simulink model "EV_Powertrain"  (R2021a)
settings: Solver=FixedStepAuto  StartTime=0.0  StopTime=993  FixedStep=0.5  RelTol=1e-3
values from neighbouring files (symbols this model uses):
  A = 3.8065    [Powertrain_Imports.m]
  B_Voltage = 364.8    [Powertrain_Imports.m]
  Ccap = 33.1    [Powertrain_Imports.m]
  Cd = 0.28    [Powertrain_Imports.m]
  Crf = 0.015    [Powertrain_Imports.m]
  Cv = 3.8    [Powertrain_Imports.m]
  Distance = 4.874    [Powertrain_Imports.m]
  GR = 7.9377    [Powertrain_Imports.m]
  GVM = M+Md    (= 1710.665)    [Powertrain_Imports.m]
  GVW = GVM*g    (= 16781.62365)    [Powertrain_Imports.m]
  ISOC = 1    [Powertrain_Imports.m]
  Neff = 0.89    [Powertrain_Imports.m]
  rho = 1.225    [Powertrain_Imports.m]
  Rw = 0.2032    [Powertrain_Imports.m]
undefined symbols (not defined in the file or in its folder): Motor_controller_eff, Motor_controller_reff, Motor_eff, Motor_reff
settings Model: Creator=mluser  LastModifiedBy=mluser

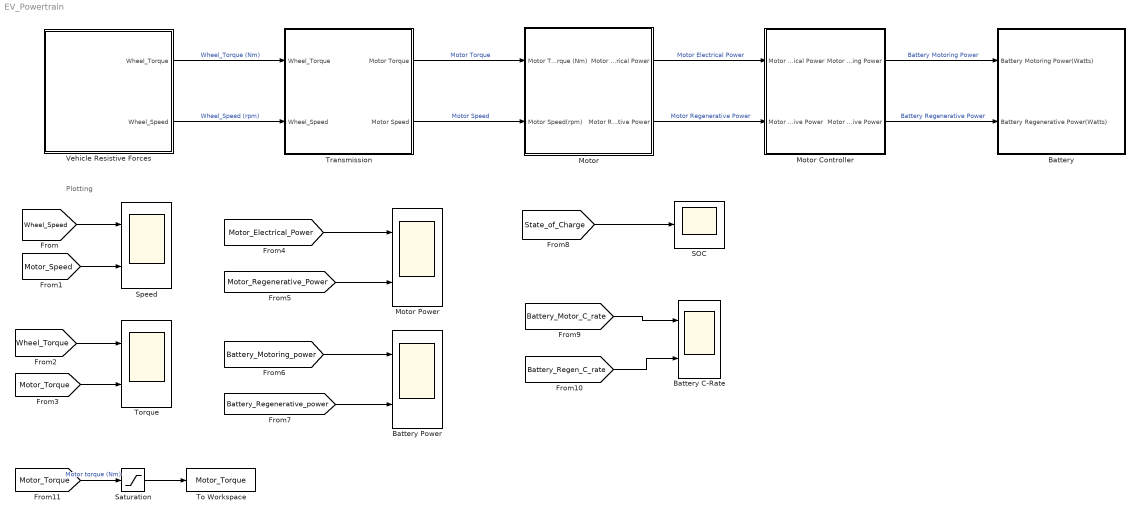
== system EV_Powertrain ==
  note: Plotting
  Battery : Subsystem
  Battery C-Rate : Scope  NumInputPorts=2
  Battery Power : Scope  NumInputPorts=2
  Motor : Subsystem
  Motor Controller : Subsystem
  Motor Power : Scope  NumInputPorts=2
  SOC : Scope
  Saturation : Saturate  UpperLimit=inf  LowerLimit=0
  Speed : Scope  NumInputPorts=2
  To Workspace : ToWorkspace  VariableName=Motor_Torque  SaveFormat=Timeseries  SampleTime=-1
  Torque : Scope  NumInputPorts=2
  Transmission : Subsystem
  Vehicle Resistive Forces : Subsystem
  wires:
  Vehicle Resistive Forces/1(Wheel_Torque) -> Transmission/1(Wheel_Torque)  "Wheel_Torque (Nm)"
  Vehicle Resistive Forces/2(Wheel_Speed) -> Transmission/2(Wheel_Speed)  "Wheel_Speed (rpm)"
  [Wheel_Speed] -> Speed/1
  [Motor_Speed] -> Speed/2
  [Motor_Torque] -> Torque/2
  [Wheel_Torque] -> Torque/1
  Transmission/1(Motor Torque) -> Motor/1(Motor Torque (Nm))  "Motor Torque"
  Transmission/2(Motor Speed) -> Motor/2(Motor Speed(rpm))  "Motor Speed"
  [Motor_Electrical_Power] -> Motor Power/1
  [Motor_Regenerative_Power] -> Motor Power/2
  Motor/1(Motor Electrical Power) -> Motor Controller/1(Motor Electrical Power)  "Motor Electrical Power"
  Motor/2(Motor Regenerative Power) -> Motor Controller/2(Motor Regenerative Power)  "Motor Regenerative Power"
  [Battery_Motoring_power] -> Battery Power/1
  [Battery_Regenerative_power] -> Battery Power/2
  Motor Controller/1(Motor Controller Motoring Power) -> Battery/1(Battery Motoring Power(Watts))  "Battery Motoring Power"
  Motor Controller/2(Motor Controller Regenerative Power) -> Battery/2(Battery Regenerative Power(Watts))  "Battery Regenerative Power"
  [State_of_Charge] -> SOC/1
  [Battery_Regen_C_rate] -> Battery C-Rate/2
  [Battery_Motor_C_rate] -> Battery C-Rate/1
  [Motor_Torque] -> Saturation/1  "Motor torque (Nm)"
  Saturation/1 -> To Workspace/1

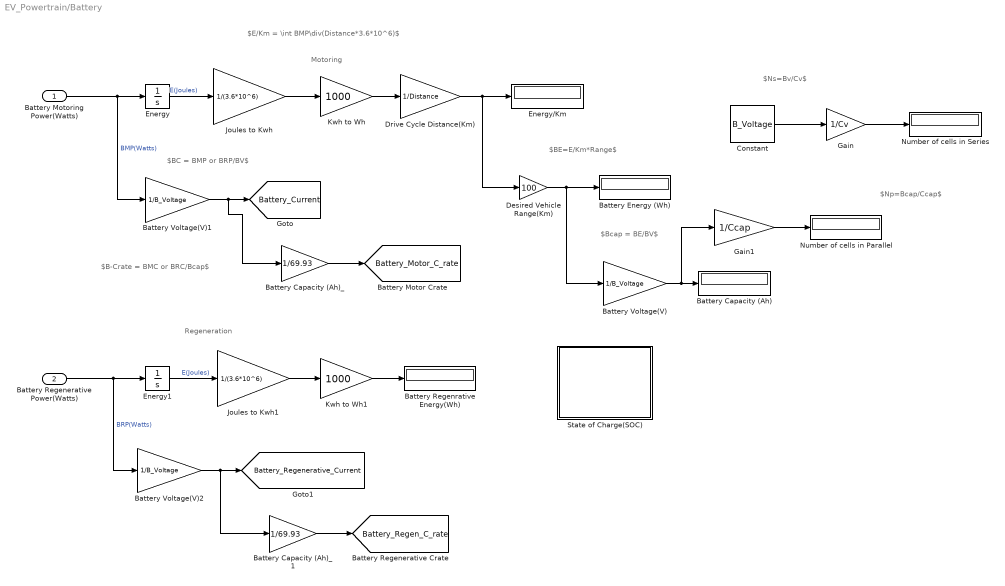
== system EV_Powertrain/Battery ==
  note: $Np=Bcap/Ccap$
  note: $Ns=Bv/Cv$
  note: Regeneration
  note: $B-Crate = BMC or BRC/Bcap$
  note: $BC = BMP or BRP/BV$
  note: $Bcap = BE/BV$
  note: $BE=E/Km*Range$
  note: $E/Km = \int BMP\div(Distance*3.6*10^6)$
  note: Motoring
  Battery Motoring Power(Watts) : Inport
  Battery Regenerative Power(Watts) : Inport  Port=2
  Battery Regenrative Energy(Wh) : Display
  Battery Capacity (Ah) : Display
  Battery Capacity (Ah)_ : Gain  Gain=1/69.93
  Battery Capacity (Ah)_1 : Gain  Gain=1/69.93
  Battery Energy (Wh) : Display
  Battery Voltage(V) : Gain  Gain=1/B_Voltage
  Battery Voltage(V)1 : Gain  Gain=1/B_Voltage
  Battery Voltage(V)2 : Gain  Gain=1/B_Voltage
  Constant : Constant  Value=B_Voltage
  Desired Vehicle Range(Km) : Gain  Gain=100
  Drive Cycle Distance(Km) : Gain  Gain=1/Distance
  Energy : Integrator
  Energy/Km : Display
  Energy1 : Integrator
  Gain : Gain  Gain=1/Cv
  Gain1 : Gain  Gain=1/Ccap
  Joules to Kwh : Gain  Gain=1/(3.6*10^6)
  Joules to Kwh1 : Gain  Gain=1/(3.6*10^6)
  Kwh to Wh : Gain  Gain=1000
  Kwh to Wh1 : Gain  Gain=1000
  Number of cells in Parallel : Display
  Number of cells in Series : Display
  State of Charge(SOC) : Subsystem
  tag scope: Battery_Current=global, Battery_Motor_C_rate=global, Battery_Regen_C_rate=global, Battery_Regenerative_Current=global
  wires:
  Battery Motoring Power(Watts)/1 -> Battery Voltage(V)1/1, Energy/1  "BMP(Watts)"
  Kwh to Wh/1 -> Drive Cycle Distance(Km)/1
  Joules to Kwh/1 -> Kwh to Wh/1
  Energy/1 -> Joules to Kwh/1  "E(Joules)"
  Drive Cycle Distance(Km)/1 -> Desired Vehicle Range(Km)/1, Energy/Km/1
  Desired Vehicle Range(Km)/1 -> Battery Voltage(V)/1, Battery Energy (Wh)/1
  Battery Voltage(V)/1 -> Gain1/1, Battery Capacity (Ah)/1
  Battery Voltage(V)1/1 -> Battery Capacity (Ah)_/1, [Battery_Current]
  Battery Voltage(V)2/1 -> Battery Capacity (Ah)_1/1, [Battery_Regenerative_Current]
  Battery Regenerative Power(Watts)/1 -> Battery Voltage(V)2/1, Energy1/1  "BRP(Watts)"
  Energy1/1 -> Joules to Kwh1/1  "E(Joules)"
  Joules to Kwh1/1 -> Kwh to Wh1/1
  Kwh to Wh1/1 -> Battery Regenrative Energy(Wh)/1
  Battery Capacity (Ah)_/1 -> [Battery_Motor_C_rate]
  Battery Capacity (Ah)_1/1 -> [Battery_Regen_C_rate]
  Constant/1 -> Gain/1
  Gain/1 -> Number of cells in Series/1
  Gain1/1 -> Number of cells in Parallel/1

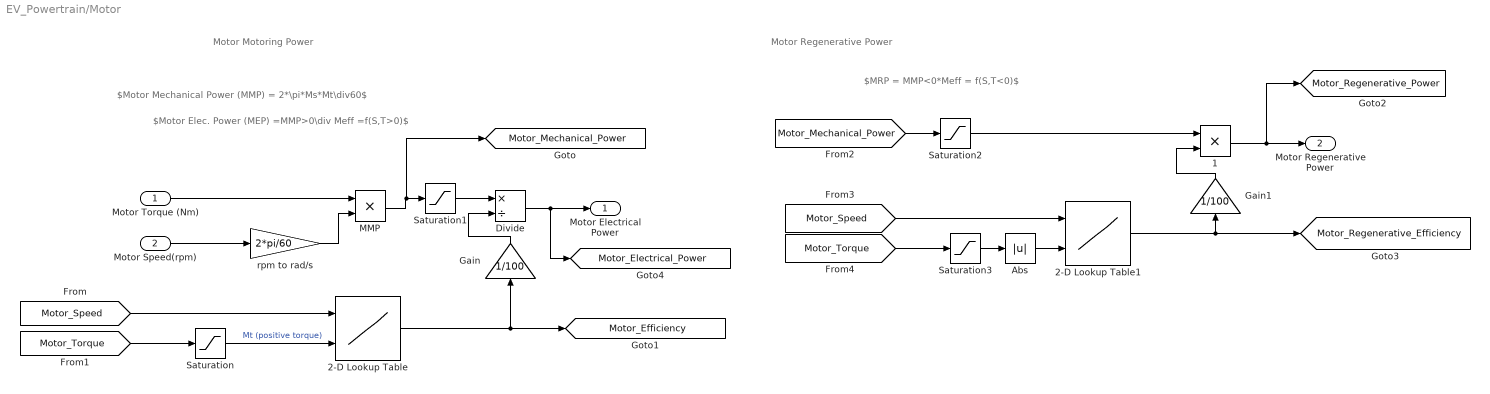
== system EV_Powertrain/Motor ==
  note: $MRP = MMP<0*Meff = f(S,T<0)$
  note: Motor Motoring Power
  note: $Motor Elec. Power (MEP) =MMP>0\div Meff =f(S,T>0)$
  note: $Motor Mechanical Power (MMP) = 2*\pi*Ms*Mt\div60$
  note: Motor Regenerative Power
  Motor Torque (Nm) : Inport
  Motor Speed(rpm) : Inport  Port=2
  1 : Product
  2-D Lookup Table : Lookup_n-D  BreakpointsForDimension1=Motor_eff.Speed  BreakpointsForDimension2=Motor_eff.Torque  Table=Motor_eff.eff  InternalRulePriority=Speed  RndMeth=Simplest  InputSameDT=on
      settings: InputPortMap=u0,u1
  2-D Lookup Table1 : Lookup_n-D  BreakpointsForDimension1=Motor_reff.Speed  BreakpointsForDimension2=Motor_reff.Torque  Table=Motor_reff.eff  InternalRulePriority=Speed  RndMeth=Simplest  InputSameDT=on
      settings: InputPortMap=u0,u1
  Abs : Abs
  Divide : Product  Inputs=*/
  Gain : Gain  Gain=1/100
  Gain1 : Gain  Gain=1/100
  MMP : Product
  Saturation : Saturate  UpperLimit=inf  LowerLimit=0
  Saturation1 : Saturate  UpperLimit=inf  LowerLimit=0
  Saturation2 : Saturate  UpperLimit=0  LowerLimit=-inf
  Saturation3 : Saturate  UpperLimit=0  LowerLimit=-inf
  rpm to rad/s : Gain  Gain=2*pi/60
  Motor Electrical Power : Outport
  Motor Regenerative Power : Outport  Port=2
  tag scope: Motor_Efficiency=global, Motor_Electrical_Power=global, Motor_Mechanical_Power=global, Motor_Regenerative_Efficiency=global, Motor_Regenerative_Power=global
  wires:
  Motor Speed(rpm)/1 -> rpm to rad/s/1
  Motor Torque (Nm)/1 -> MMP/1
  rpm to rad/s/1 -> MMP/2
  [Motor_Torque] -> Saturation/1
  Saturation/1 -> 2-D Lookup Table/2  "Mt (positive torque)"
  [Motor_Speed] -> 2-D Lookup Table/1
  Gain/1 -> Divide/2
  Divide/1 -> [Motor_Electrical_Power], Motor Electrical Power/1
  2-D Lookup Table/1 -> [Motor_Efficiency], Gain/1
  MMP/1 -> [Motor_Mechanical_Power], Saturation1/1
  Saturation1/1 -> Divide/1
  [Motor_Mechanical_Power] -> Saturation2/1
  [Motor_Torque] -> Saturation3/1
  [Motor_Speed] -> 2-D Lookup Table1/1
  Saturation3/1 -> Abs/1
  Abs/1 -> 2-D Lookup Table1/2
  1/1 -> [Motor_Regenerative_Power], Motor Regenerative Power/1
  Saturation2/1 -> 1/1
  2-D Lookup Table1/1 -> [Motor_Regenerative_Efficiency], Gain1/1
  Gain1/1 -> 1/2

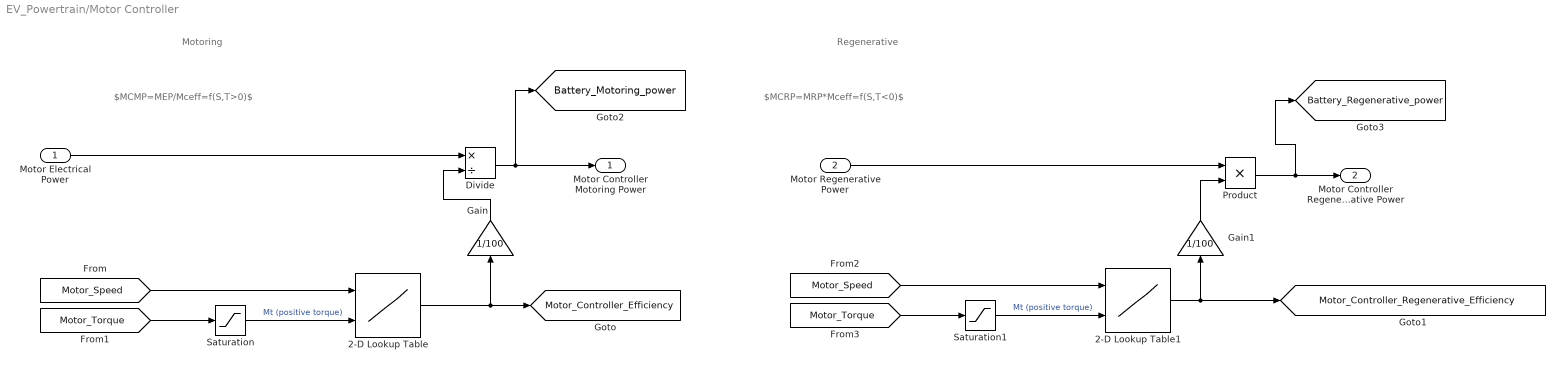
== system EV_Powertrain/Motor Controller ==
  note: Motoring
  note: $MCMP=MEP/Mceff=f(S,T>0)$
  note: Regenerative
  note: $MCRP=MRP*Mceff=f(S,T<0)$
  Motor Electrical Power : Inport
  Motor Regenerative Power : Inport  Port=2
  2-D Lookup Table : Lookup_n-D  BreakpointsForDimension1=Motor_controller_eff.Speed  BreakpointsForDimension2=Motor_controller_eff.Torque  Table=Motor_controller_eff.eff  InternalRulePriority=Speed  RndMeth=Simplest  InputSameDT=on
      settings: InputPortMap=u0,u1
  2-D Lookup Table1 : Lookup_n-D  BreakpointsForDimension1=Motor_controller_reff.Speed  BreakpointsForDimension2=Motor_controller_reff.Torque  Table=Motor_controller_reff.eff  InternalRulePriority=Speed  RndMeth=Simplest  InputSameDT=on
      settings: InputPortMap=u0,u1
  Divide : Product  Inputs=*/
  Gain : Gain  Gain=1/100
  Gain1 : Gain  Gain=1/100
  Product : Product
  Saturation : Saturate  UpperLimit=inf  LowerLimit=0
  Saturation1 : Saturate  UpperLimit=0  LowerLimit=-inf
  Motor Controller Motoring Power : Outport
  Motor Controller Regenerative Power : Outport  Port=2
  tag scope: Battery_Motoring_power=global, Battery_Regenerative_power=global, Motor_Controller_Efficiency=global, Motor_Controller_Regenerative_Efficiency=global
  wires:
  2-D Lookup Table/1 -> Gain/1, [Motor_Controller_Efficiency]
  [Motor_Speed] -> 2-D Lookup Table/1
  Saturation/1 -> 2-D Lookup Table/2  "Mt (positive torque)"
  [Motor_Torque] -> Saturation/1
  Gain/1 -> Divide/2
  Motor Electrical Power/1 -> Divide/1
  Divide/1 -> Motor Controller Motoring Power/1, [Battery_Motoring_power]
  [Motor_Speed] -> 2-D Lookup Table1/1
  2-D Lookup Table1/1 -> [Motor_Controller_Regenerative_Efficiency], Gain1/1
  Saturation1/1 -> 2-D Lookup Table1/2  "Mt (positive torque)"
  [Motor_Torque] -> Saturation1/1
  Gain1/1 -> Product/2
  Motor Regenerative Power/1 -> Product/1
  Product/1 -> [Battery_Regenerative_power], Motor Controller Regenerative Power/1

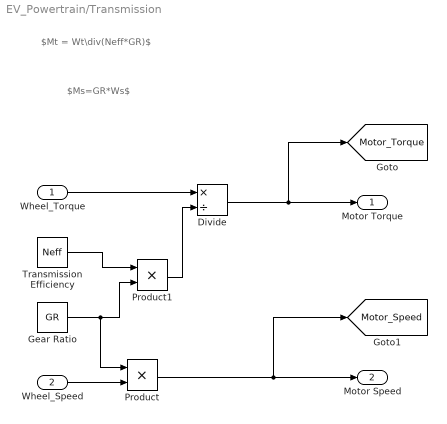
== system EV_Powertrain/Transmission ==
  note: $Mt = Wt\div(Neff*GR)$
  note: $Ms=GR*Ws$
  Wheel_Torque : Inport
  Wheel_Speed : Inport  Port=2
  Divide : Product  Inputs=*/
  Gear Ratio : Constant  Value=GR
  Product : Product
  Product1 : Product
  Transmission Efficiency : Constant  Value=Neff
  Motor Torque : Outport
  Motor Speed : Outport  Port=2
  tag scope: Motor_Speed=global, Motor_Torque=global
  wires:
  Gear Ratio/1 -> Product1/2, Product/1
  Wheel_Speed/1 -> Product/2
  Product/1 -> [Motor_Speed], Motor Speed/1
  Transmission Efficiency/1 -> Product1/1
  Wheel_Torque/1 -> Divide/1
  Product1/1 -> Divide/2
  Divide/1 -> [Motor_Torque], Motor Torque/1

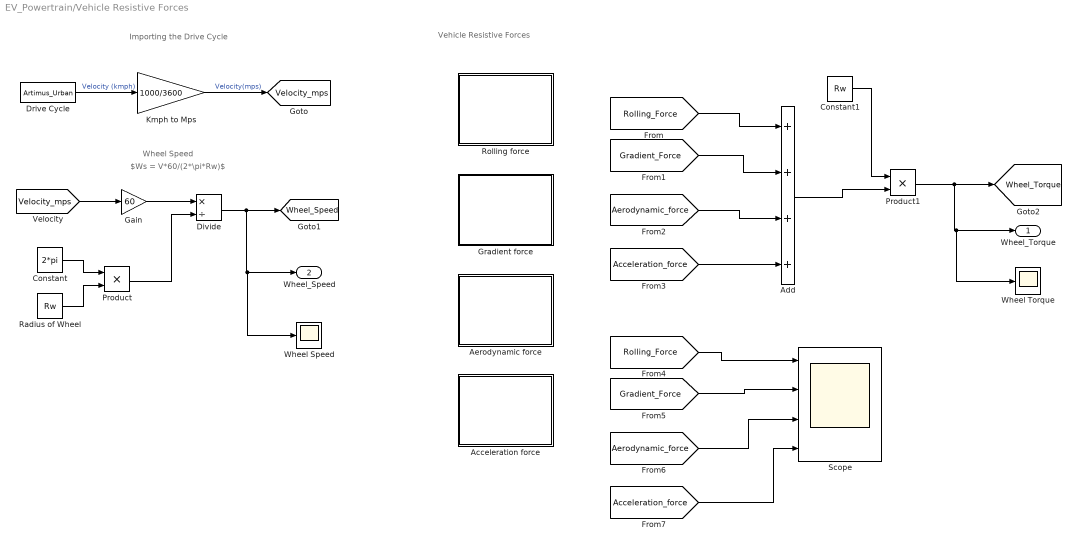
== system EV_Powertrain/Vehicle Resistive Forces ==
  note: Vehicle Resistive Forces
  note: $Ws = V*60/(2*\pi*Rw)$
  note: Wheel Speed
  note: Importing the Drive Cycle
  Acceleration force : Subsystem
  Add : Sum  Inputs=++++
  Aerodynamic force : Subsystem
  Constant : Constant  Value=2*pi
  Constant1 : Constant  Value=Rw
  Divide : Product  Inputs=*/
  Drive Cycle : FromWorkspace  VariableName=Artimus_Urban
  Gain : Gain  Gain=60
  Gradient force : Subsystem
  Kmph to Mps : Gain  Gain=1000/3600
  Product : Product
  Product1 : Product
  Radius of Wheel : Constant  Value=Rw
  Rolling force : Subsystem
  Scope : Scope  NumInputPorts=4
  Wheel Speed : Scope
  Wheel Torque : Scope
  Wheel_Torque : Outport
  Wheel_Speed : Outport  Port=2
  tag scope: Velocity_mps=global, Wheel_Speed=global, Wheel_Torque=global
  wires:
  Drive Cycle/1 -> Kmph to Mps/1  "Velocity (kmph)"
  Kmph to Mps/1 -> [Velocity_mps]  "Velocity(mps)"
  [Velocity_mps] -> Gain/1
  Constant/1 -> Product/1
  Radius of Wheel/1 -> Product/2
  Gain/1 -> Divide/1
  Product/1 -> Divide/2
  Divide/1 -> Wheel Speed/1, Wheel_Speed/1, [Wheel_Speed]
  [Rolling_Force] -> Add/1
  [Gradient_Force] -> Add/2
  [Aerodynamic_force] -> Add/3
  [Acceleration_force] -> Add/4
  Add/1 -> Product1/2
  Constant1/1 -> Product1/1
  Product1/1 -> Wheel Torque/1, Wheel_Torque/1, [Wheel_Torque]
  [Rolling_Force] -> Scope/1
  [Gradient_Force] -> Scope/2
  [Aerodynamic_force] -> Scope/3
  [Acceleration_force] -> Scope/4

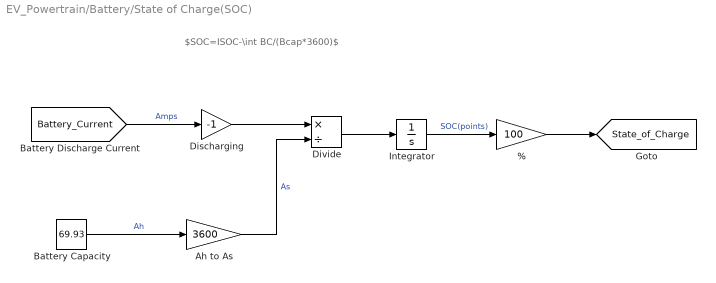
== system EV_Powertrain/Battery/State of Charge(SOC) ==
  note: $SOC=ISOC-\int BC/(Bcap*3600)$
  % : Gain  Gain=100
  Ah to As : Gain  Gain=3600
  Battery Capacity : Constant  Value=69.93
  Discharging : Gain  Gain=-1
  Divide : Product  Inputs=*/
  Integrator : Integrator  InitialCondition=ISOC
  tag scope: State_of_Charge=global
  wires:
  [Battery_Current] -> Discharging/1  "Amps"
  Battery Capacity/1 -> Ah to As/1  "Ah"
  Ah to As/1 -> Divide/2  "As"
  Discharging/1 -> Divide/1
  Divide/1 -> Integrator/1
  Integrator/1 -> %/1  "SOC(points)"
  %/1 -> [State_of_Charge]

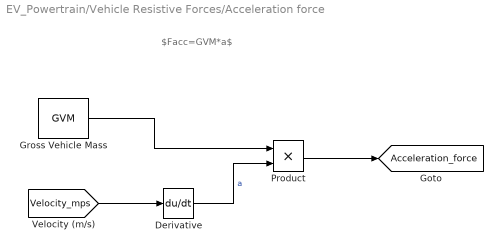
== system EV_Powertrain/Vehicle Resistive Forces/Acceleration force ==
  note: $Facc=GVM*a$
  Derivative : Derivative
  Gross Vehicle Mass : Constant  Value=GVM
  Product : Product
  tag scope: Acceleration_force=global
  wires:
  [Velocity_mps] -> Derivative/1
  Gross Vehicle Mass/1 -> Product/1
  Derivative/1 -> Product/2  "a"
  Product/1 -> [Acceleration_force]

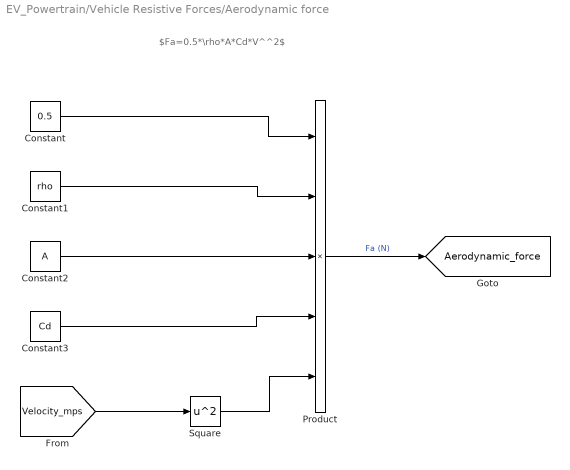
== system EV_Powertrain/Vehicle Resistive Forces/Aerodynamic force ==
  note: $Fa=0.5*\rho*A*Cd*V^^2$
  Constant : Constant  Value=0.5
  Constant1 : Constant  Value=rho
  Constant2 : Constant  Value=A
  Constant3 : Constant  Value=Cd
  Product : Product  Inputs=5
  Square : Math  Operator=square  SaturateOnIntegerOverflow=on
  tag scope: Aerodynamic_force=global
  wires:
  [Velocity_mps] -> Square/1
  Square/1 -> Product/5
  Constant3/1 -> Product/4
  Constant2/1 -> Product/3
  Constant1/1 -> Product/2
  Constant/1 -> Product/1
  Product/1 -> [Aerodynamic_force]  "Fa (N)"

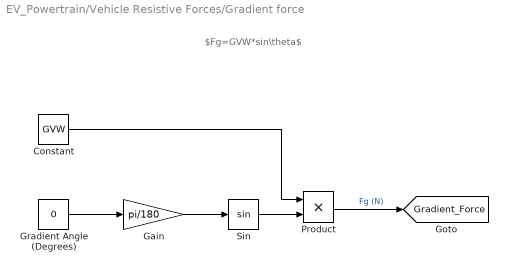
== system EV_Powertrain/Vehicle Resistive Forces/Gradient force ==
  note: $Fg=GVW*sin\theta$
  Constant : Constant  Value=GVW
  Gain : Gain  Gain=pi/180
  Gradient Angle (Degrees) : Constant  Value=0
  Product : Product
  Sin : Trigonometry
  tag scope: Gradient_Force=global
  wires:
  Gain/1 -> Sin/1
  Gradient Angle (Degrees)/1 -> Gain/1
  Constant/1 -> Product/1
  Sin/1 -> Product/2
  Product/1 -> [Gradient_Force]  "Fg (N)"

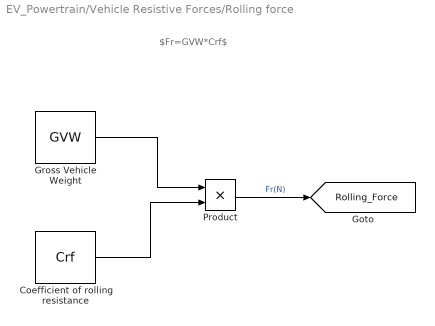
== system EV_Powertrain/Vehicle Resistive Forces/Rolling force ==
  note: $Fr=GVW*Crf$
  Coefficient of rolling resistance : Constant  Value=Crf
  Gross Vehicle Weight : Constant  Value=GVW
  Product : Product
  tag scope: Rolling_Force=global
  wires:
  Gross Vehicle Weight/1 -> Product/1
  Coefficient of rolling resistance/1 -> Product/2
  Product/1 -> [Rolling_Force]  "Fr(N)"
